simulink model "TBRe19_ECU_1_WORKING_190726"  (R2017b)
settings: Solver=FixedStepDiscrete  StartTime=0.0  StopTime=inf  FixedStep=0.0001  RelTol=1e-3
PostLoadFcn:
  | model_init();
libraries: simulink x17
(part 6 of 7)

== system TBRe19_ECU_1_WORKING_190726/MainTask/Pre_Processing_Layer/Pedal_Box/APPS and BP Plausibility ==
  note: Invert the logic so that if error is active, throttle gets multiplied by zero
  note: This block outputs the previous state from previous sample
  note: Note: This is needed by rules - including specified percentages
  note: If brake is above 20% AND accelerator is above 25%, then hold the error on until throttle is less than 5%
  note: If accelerator and brake pedal are pressed at the same time, then wait for both pedals to return to zero before sending further torque requests
  note: function [Throttle_Percentage, APPS_BP_Implausibility] = APPS_BP_Plausibility_Check(Throttle_In, Brake_In, APPS_BP_Implausibility_Prv)
      | %Plausibility check on both throttle and brake
      |
      | %Implausible case: when both brake and throttle applied
      | if (Brake_In >=20 && Throttle_In > 25)
      |     APPS_BP_Implausibility = true;
      |     Throttle_Percentage =uint8(0);
      |
      | %Implausible case: when brake pressed but throttle still not below 5%
      | elseif (APPS_BP_Implausibility_Prv && Throttle_In > 5)
      |     APPS_BP_Implausibility = true;
      |     Throttle_Percentage =uint8(0);
      |
      | %Plausible case, throttle goes below 5%
      | elseif (APPS_BP_Implausibility_Prv && Throttle_In < 5)
      |     APPS_BP_Implausibility = false;
      |     Throttle_Percentage =uint8(Throttle_In);
      |
      | %Plausible case, normal operation
      | else
      |     APPS_BP_Implausibility = false;
      |     Throttle_Percentage =uint8(Throttle_In);
      | end
  Throttle_In : Inport
  Brake_% : Inport  Port=2
  Constant : Constant  Value=20
  Constant1 : Constant  Value=25
  Constant2 : Constant  Value=5
  Logical Operator : Logic  AllPortsSameDT=off  OutDataTypeStr=boolean
  Logical Operator1 : Logic  AllPortsSameDT=off  OutDataTypeStr=boolean
  Logical Operator2 : Logic  Operator=OR  AllPortsSameDT=off  OutDataTypeStr=boolean
  Logical Operator3 : Logic  Operator=NOT  Inputs=1  AllPortsSameDT=off  OutDataTypeStr=boolean
  Product : Product  OutDataTypeStr=uint8
  Relational Operator : RelationalOperator  OutDataTypeStr=boolean  RndMeth=Simplest
  Relational Operator1 : RelationalOperator  Operator=>  OutDataTypeStr=boolean  RndMeth=Simplest
  Relational Operator2 : RelationalOperator  Operator=>  OutDataTypeStr=boolean  RndMeth=Simplest
  prv_APPS_BP1 : Delay  DelayLength=1  InitialCondition=0
  Throttle_% : Outport
  APPS_BP_Implausibility : Outport  Port=2
  wires:
  Brake_%/1 -> Relational Operator/1
  Constant/1 -> Relational Operator/2
  Constant1/1 -> Relational Operator1/2
  Constant2/1 -> Relational Operator2/2
  Throttle_In/1 -> Product/2, Relational Operator2/1, Relational Operator1/1
  prv_APPS_BP1/1 -> Logical Operator1/2
  Relational Operator2/1 -> Logical Operator1/1
  Relational Operator/1 -> Logical Operator/1
  Relational Operator1/1 -> Logical Operator/2
  Logical Operator2/1 -> APPS_BP_Implausibility/1, Logical Operator3/1, prv_APPS_BP1/1
  Logical Operator1/1 -> Logical Operator2/2
  Logical Operator/1 -> Logical Operator2/1
  Product/1 -> Throttle_%/1
  Logical Operator3/1 -> Product/1

== system TBRe19_ECU_1_WORKING_190726/MainTask/Pre_Processing_Layer/Pedal_Box/APPS_Implausibility_Check ==
  note: This sets torque to zero if APPS implausibility happens
  note: Send to CAN bus
  note: Note: 100ms is measured using 10 delays. As task runs every 10ms, 10 delays will result in a 100ms delay
  note: If the error happens continuosly for 100ms then the throttle output should be set to zero
  note: Check to see if Throttle2 is within the range of Throttle1 +/- 15%
  note: 15% is defined in rules
  note: function [APPS_Implausbility, Throttle_Percentage] = APPS_Implausibility_Check(Pedal_Sensor_Fail, Throttle1_Per, Throttle2_Per)
      | %Limit generation for comparison
      | Upper_Limit = Throttle1_Per+15;
      | Lower_Limit = Throttle1_Per-15;
      |
      | %Passes one throttle if in range and no pedal sensor errors
      | if ((Lower_Limit <= Throttle2_Per) && (Throttle2_Per <= Upper_Limit)&& Pedal_Sensor_Fail == 0)
      |     Throttle_Percentage = uint8(max(Throttle1_Per, Throttle2_Per));
      |     APPS_Implausbility = false;
      | %All other conditions result in no throttle being applied
      | else
      |     Throttle_Percentage = uint8(0);
      |     APPS_Implausbility = true;
      | end
      |
      | end
  Throttle1_Per : Inport
  Throttle2_Per : Inport  Port=2
  Constant : Constant  Value=15
  Data Type Conversion : DataTypeConversion  OutDataTypeStr=int8
  Logical Operator : Logic  Operator=OR  AllPortsSameDT=off  OutDataTypeStr=boolean
  Logical Operator3 : Logic  Operator=NOT  Inputs=1  AllPortsSameDT=off  OutDataTypeStr=boolean
  LowerLinit : Sum  Inputs=-+
  MinMax : MinMax  Inputs=2
  Product : Product
  Product of Elements : Product  Inputs=*
  Relational Operator : RelationalOperator  OutDataTypeStr=boolean  RndMeth=Simplest
  Relational Operator1 : RelationalOperator  Operator=<=  OutDataTypeStr=boolean  RndMeth=Simplest
  Tapped Delay : simulink/Discrete/Tapped Delay  vinit=0  samptime=-1  NumDelays=10  DelayOrder=Oldest  includeCurrent=off
  UpperLinit : Sum
  APPS_Implausibility : Outport
  Throttle_% : Outport  Port=2
  wires:
  Throttle1_Per/1 -> MinMax/1, UpperLinit/1, LowerLinit/2
  Throttle2_Per/1 -> MinMax/2, Relational Operator1/1, Relational Operator/1
  Logical Operator/1 -> Tapped Delay/1  "APPS_Implausibility"
  Constant/1 -> UpperLinit/2, LowerLinit/1
  UpperLinit/1 -> Relational Operator/2
  LowerLinit/1 -> Relational Operator1/2
  Relational Operator/1 -> Logical Operator/1
  Relational Operator1/1 -> Logical Operator/2
  Logical Operator3/1 -> Data Type Conversion/1
  Data Type Conversion/1 -> Product/2
  Tapped Delay/1 -> Product of Elements/1
  Product of Elements/1 -> APPS_Implausibility/1, Logical Operator3/1
  MinMax/1 -> Product/1
  Product/1 -> Throttle_%/1

== system TBRe19_ECU_1_WORKING_190726/MainTask/Pre_Processing_Layer/Pedal_Box/BPPS_Implausibility_Check ==
  note: Note: Not needed for rules
  note: Output to CAN
  note: function [APPS_Implausbility, Throttle_Percentage] = APPS_Implausibility_Check(Pedal_Sensor_Fail, Throttle1_Per, Throttle2_Per)
      | %Limit generation for comparison
      | Upper_Limit = Throttle1_Per+15;
      | Lower_Limit = Throttle1_Per-15;
      |
      | %Passes one throttle if in range and no pedal sensor errors
      | if ((Lower_Limit <= Throttle2_Per) && (Throttle2_Per <= Upper_Limit)&& Pedal_Sensor_Fail == 0)
      |     Throttle_Percentage = uint8(max(Throttle1_Per, Throttle2_Per));
      |     APPS_Implausbility = false;
      | %All other conditions result in no throttle being applied
      | else
      |     Throttle_Percentage = uint8(0);
      |     APPS_Implausbility = true;
      | end
      |
      | end
  note: If the error happens continuosly for 100ms then the throttle output should be set to zero
  note: Note: 100ms is measured using 10 delays. As task runs every 10ms, 10 delays will result in a 100ms delay
  Brake1_Per : Inport
  Brake2_Per : Inport  Port=2
  Constant : Constant  Value=15
  Logical Operator : Logic  Operator=OR  AllPortsSameDT=off  OutDataTypeStr=boolean
  LowerLinit : Sum  Inputs=-+
  MinMax : MinMax  Function=max  Inputs=2
  Product of Elements : Product  Inputs=*
  Relational Operator : RelationalOperator  OutDataTypeStr=boolean  RndMeth=Simplest
  Relational Operator1 : RelationalOperator  Operator=<=  OutDataTypeStr=boolean  RndMeth=Simplest
  Tapped Delay : simulink/Discrete/Tapped Delay  vinit=0  samptime=-1  NumDelays=10  DelayOrder=Oldest  includeCurrent=off
  UpperLinit : Sum
  Brake_% : Outport
  BPPS_Implausibility : Outport  Port=2
  wires:
  Brake1_Per/1 -> MinMax/1, UpperLinit/1, LowerLinit/2
  Brake2_Per/1 -> MinMax/2, Relational Operator1/1, Relational Operator/1
  Logical Operator/1 -> Tapped Delay/1  "APPS_Implausibility"
  Constant/1 -> UpperLinit/2, LowerLinit/1
  UpperLinit/1 -> Relational Operator/2
  LowerLinit/1 -> Relational Operator1/2
  Relational Operator/1 -> Logical Operator/1
  Relational Operator1/1 -> Logical Operator/2
  Tapped Delay/1 -> Product of Elements/1
  Product of Elements/1 -> BPPS_Implausibility/1
  MinMax/1 -> Brake_%/1

== system TBRe19_ECU_1_WORKING_190726/MainTask/Pre_Processing_Layer/Pedal_Box/Sensor Plausibility ==
  note: Check if the readings from the sensors are outside expected range
      | e.g. If a 5V sensor is giving a reading of 12V
      |
      | Note: Not needed for rules
  <Throttle1_Voltage> : Inport
  <Throttle2_Voltage> : Inport  Port=2
  <Brake_Voltage> : Inport  Port=3
  <Brake_Voltage>1 : Inport  Port=4
  <Brake_Voltage>2 : Inport  Port=5
  Sensor_Diag : MATLAB Function  TreatAsAtomicUnit=on
  Pedal_Sensor_Fail : Outport
  TV1_Out : Outport  Port=2
  TV2_Out : Outport  Port=3
  BVPot_Out : Outport  Port=4
  BV1_Out : Outport  Port=5
  BV1_Out1 : Outport  Port=6
  wires:
  <Throttle1_Voltage>/1 -> Sensor_Diag/1(TV_1)
  <Throttle2_Voltage>/1 -> Sensor_Diag/2(TV_2)
  <Brake_Voltage>/1 -> Sensor_Diag/3(BV_POT)
  Sensor_Diag/1(Pedal_Sensor_Fail) -> Pedal_Sensor_Fail/1
  Sensor_Diag/2(TV1_Out) -> TV1_Out/1
  Sensor_Diag/3(TV2_Out) -> TV2_Out/1
  Sensor_Diag/4(BVPot_Out) -> BVPot_Out/1
  <Brake_Voltage>1/1 -> Sensor_Diag/4(BV_1)
  <Brake_Voltage>2/1 -> Sensor_Diag/5(BV_2)
  Sensor_Diag/5(BV1_Out) -> BV1_Out/1
  Sensor_Diag/6(BV2_Out) -> BV1_Out1/1

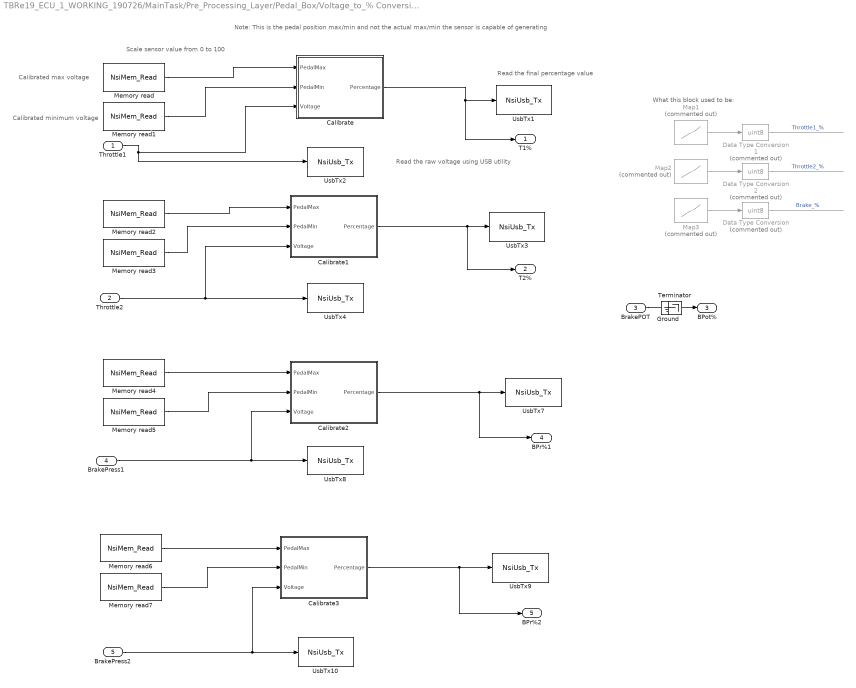
== system TBRe19_ECU_1_WORKING_190726/MainTask/Pre_Processing_Layer/Pedal_Box/Voltage_to_% Conversion ==
  note: Read the final percentage value
  note: Read the raw voltage using USB utility
  note: Note: This is the pedal position max/min and not the actual max/min the sensor is capable of generating
  note: Calibrated minimum voltage
  note: Calibrated max voltage
  note: What this block used to be:
  note: Scale sensor value from 0 to 100
  Throttle1 : Inport
  Throttle2 : Inport  Port=2
  BrakePOT : Inport  Port=3
  BrakePress1 : Inport  Port=4
  BrakePress2 : Inport  Port=5
  Calibrate : Subsystem
  Calibrate1 : Subsystem
  Calibrate2 : Subsystem
  Calibrate3 : Subsystem
  Data Type Conversion : DataTypeConversion  Commented=on  OutDataTypeStr=uint8
  Data Type Conversion1 : DataTypeConversion  Commented=on  OutDataTypeStr=uint8
  Data Type Conversion2 : DataTypeConversion  Commented=on  OutDataTypeStr=uint8
  Ground : Ground
  Map1 : Lookup_n-D  Commented=on  NumberOfTableDimensions=1  BreakpointsForDimension1=[0000,5000]  Table=[0,100]  ExtrapMethod=Clip  UseLastTableValue=on  InternalRulePriority=Speed  RndMeth=Simplest  InputSameDT=on
  Map2 : Lookup_n-D  Commented=on  NumberOfTableDimensions=1  BreakpointsForDimension1=[0000,5000]  Table=[0,100]  ExtrapMethod=Clip  UseLastTableValue=on  InternalRulePriority=Speed  RndMeth=Simplest  InputSameDT=on
  Map3 : Lookup_n-D  Commented=on  NumberOfTableDimensions=1  BreakpointsForDimension1=[2800,5600]  Table=[0,100]  ExtrapMethod=Clip  UseLastTableValue=on  InternalRulePriority=Speed  RndMeth=Simplest  InputSameDT=on
  Memory read : S-Function  FunctionName=NsiMem_Read  Parameters=name_var,type_var,size_var,tunable_var  SFunctionDeploymentMode=off  EnableBusSupport=off  mask(Memory read){name_var=Throttle1_High, type_var=Unsigned Word, size_var=1, tunable_var=on}
      mask prompts: name_var "Variable name :"; type_var "Type :"; size_var "Dim of table :"; tunable_var "Is Tunable By USB?"
      mask help: Reads current value of variable memory declared in the configurator block in calibration page.
      mask init:
      | NsiMem_Read_InitializationFcn();
      settings: OpenFcn=NsiMem_Read_OpenFcn();
      mask Help:
      | eval('block=get_param(gcb, ''RTWdata'');')
      | web([docroot '\toolbox\MUXlink\html\blocks/' block.MUXlink_BlockType '.html'])
      mask TypeOptions name_var: Gearing_Ratio | Wheel_Size | Brake1_High | Brake2_High | Throttle1_High | Throttle2_High | Brake1_Low | Brake2_Low | Throttle1_Low | Throttle2_Low | Max_Torque_Std | Max_Torque_Boost | MCU_Ignition | LV_Low_Voltage_Warning | MCUMotor_Temp_Warning | Target_Slip_Ratio | TC_P_Gain | MinTC_Torque | Max_Regen | Throttle_Active_Threshold | Brake_Active_Threshold | INV_Torque_limit | INV_Speed_Limit_Fwd | INV_Speed_limit_Rev | INV_DC_Link_Target | INV_DC_Link_Regen_Imax | INV_DC_Link_Discharge_Imax | INV_Regen_Torque_Limit | INV_Id_Debug | INV_Iq_debug | Init_System_Start | Init_System_end | Brake1_Pressure_Scaling | Brake2_Pressure_Scaling
      mask Callback name_var: NsiMem_Read_ApplyFcn(1);
      mask TypeOptions type_var: Boolean | Signed Byte | Unsigned Byte | Signed Word | Unsigned Word | Signed Double Word | Unsigned Double Word | Single Float | Double Float
      mask Callback type_var: NsiMem_Read_ApplyFcn(2);
      mask Callback size_var: NsiMem_Read_ApplyFcn(3);
      mask Callback tunable_var: NsiMem_Read_ApplyFcn(4);
      mask Display: image(imread('nsi.bmp'));text(0.5, 0.35, 'Throttle1_High', 'horizontalAlignment', 'center', 'verticalAlignment', 'base');plot([0.05 0.05 0.05 0.05 0.05 0.05 0.05 0.05 0.05 0.05]);port_label('output', 1, 'Read');
  Memory read1 : S-Function  FunctionName=NsiMem_Read  Parameters=name_var,type_var,size_var,tunable_var  SFunctionDeploymentMode=off  EnableBusSupport=off  mask(Memory read){name_var=Throttle1_Low, type_var=Unsigned Word, size_var=1, tunable_var=on}
      mask prompts: name_var "Variable name :"; type_var "Type :"; size_var "Dim of table :"; tunable_var "Is Tunable By USB?"
      mask help: Reads current value of variable memory declared in the configurator block in calibration page.
      mask init:
      | NsiMem_Read_InitializationFcn();
      settings: OpenFcn=NsiMem_Read_OpenFcn();
      mask Help:
      | eval('block=get_param(gcb, ''RTWdata'');')
      | web([docroot '\toolbox\MUXlink\html\blocks/' block.MUXlink_BlockType '.html'])
      mask TypeOptions name_var: Gearing_Ratio | Wheel_Size | Brake1_High | Brake2_High | Throttle1_High | Throttle2_High | Brake1_Low | Brake2_Low | Throttle1_Low | Throttle2_Low | Max_Torque_Std | Max_Torque_Boost | MCU_Ignition | LV_Low_Voltage_Warning | MCUMotor_Temp_Warning | Target_Slip_Ratio | TC_P_Gain | MinTC_Torque | Max_Regen | Throttle_Active_Threshold | Brake_Active_Threshold | INV_Torque_limit | INV_Speed_Limit_Fwd | INV_Speed_limit_Rev | INV_DC_Link_Target | INV_DC_Link_Regen_Imax | INV_DC_Link_Discharge_Imax | INV_Regen_Torque_Limit | INV_Id_Debug | INV_Iq_debug | Init_System_Start | Init_System_end | Brake1_Pressure_Scaling | Brake2_Pressure_Scaling
      mask Callback name_var: NsiMem_Read_ApplyFcn(1);
      mask TypeOptions type_var: Boolean | Signed Byte | Unsigned Byte | Signed Word | Unsigned Word | Signed Double Word | Unsigned Double Word | Single Float | Double Float
      mask Callback type_var: NsiMem_Read_ApplyFcn(2);
      mask Callback size_var: NsiMem_Read_ApplyFcn(3);
      mask Callback tunable_var: NsiMem_Read_ApplyFcn(4);
      mask Display: image(imread('nsi.bmp'));text(0.5, 0.35, 'Throttle1_Low', 'horizontalAlignment', 'center', 'verticalAlignment', 'base');plot([0.05 0.05 0.05 0.05 0.05 0.05 0.05 0.05 0.05 0.05]);port_label('output', 1, 'Read');
  Memory read2 : S-Function  FunctionName=NsiMem_Read  Parameters=name_var,type_var,size_var,tunable_var  SFunctionDeploymentMode=off  EnableBusSupport=off  mask(Memory read){name_var=Throttle2_High, type_var=Unsigned Word, size_var=1, tunable_var=on}
      mask prompts: name_var "Variable name :"; type_var "Type :"; size_var "Dim of table :"; tunable_var "Is Tunable By USB?"
      mask help: Reads current value of variable memory declared in the configurator block in calibration page.
      mask init:
      | NsiMem_Read_InitializationFcn();
      settings: OpenFcn=NsiMem_Read_OpenFcn();
      mask Help:
      | eval('block=get_param(gcb, ''RTWdata'');')
      | web([docroot '\toolbox\MUXlink\html\blocks/' block.MUXlink_BlockType '.html'])
      mask TypeOptions name_var: Gearing_Ratio | Wheel_Size | Brake1_High | Brake2_High | Throttle1_High | Throttle2_High | Brake1_Low | Brake2_Low | Throttle1_Low | Throttle2_Low | Max_Torque_Std | Max_Torque_Boost | MCU_Ignition | LV_Low_Voltage_Warning | MCUMotor_Temp_Warning | Target_Slip_Ratio | TC_P_Gain | MinTC_Torque | Max_Regen | Throttle_Active_Threshold | Brake_Active_Threshold | INV_Torque_limit | INV_Speed_Limit_Fwd | INV_Speed_limit_Rev | INV_DC_Link_Target | INV_DC_Link_Regen_Imax | INV_DC_Link_Discharge_Imax | INV_Regen_Torque_Limit | INV_Id_Debug | INV_Iq_debug | Init_System_Start | Init_System_end | Brake1_Pressure_Scaling | Brake2_Pressure_Scaling
      mask Callback name_var: NsiMem_Read_ApplyFcn(1);
      mask TypeOptions type_var: Boolean | Signed Byte | Unsigned Byte | Signed Word | Unsigned Word | Signed Double Word | Unsigned Double Word | Single Float | Double Float
      mask Callback type_var: NsiMem_Read_ApplyFcn(2);
      mask Callback size_var: NsiMem_Read_ApplyFcn(3);
      mask Callback tunable_var: NsiMem_Read_ApplyFcn(4);
      mask Display: image(imread('nsi.bmp'));text(0.5, 0.35, 'Throttle2_High', 'horizontalAlignment', 'center', 'verticalAlignment', 'base');plot([0.05 0.05 0.05 0.05 0.05 0.05 0.05 0.05 0.05 0.05]);port_label('output', 1, 'Read');
  Memory read3 : S-Function  FunctionName=NsiMem_Read  Parameters=name_var,type_var,size_var,tunable_var  SFunctionDeploymentMode=off  EnableBusSupport=off  mask(Memory read){name_var=Throttle2_Low, type_var=Unsigned Word, size_var=1, tunable_var=on}
      mask prompts: name_var "Variable name :"; type_var "Type :"; size_var "Dim of table :"; tunable_var "Is Tunable By USB?"
      mask help: Reads current value of variable memory declared in the configurator block in calibration page.
      mask init:
      | NsiMem_Read_InitializationFcn();
      settings: OpenFcn=NsiMem_Read_OpenFcn();
      mask Help:
      | eval('block=get_param(gcb, ''RTWdata'');')
      | web([docroot '\toolbox\MUXlink\html\blocks/' block.MUXlink_BlockType '.html'])
      mask TypeOptions name_var: Gearing_Ratio | Wheel_Size | Brake1_High | Brake2_High | Throttle1_High | Throttle2_High | Brake1_Low | Brake2_Low | Throttle1_Low | Throttle2_Low | Max_Torque_Std | Max_Torque_Boost | MCU_Ignition | LV_Low_Voltage_Warning | MCUMotor_Temp_Warning | Target_Slip_Ratio | TC_P_Gain | MinTC_Torque | Max_Regen | Throttle_Active_Threshold | Brake_Active_Threshold | INV_Torque_limit | INV_Speed_Limit_Fwd | INV_Speed_limit_Rev | INV_DC_Link_Target | INV_DC_Link_Regen_Imax | INV_DC_Link_Discharge_Imax | INV_Regen_Torque_Limit | INV_Id_Debug | INV_Iq_debug | Init_System_Start | Init_System_end | Brake1_Pressure_Scaling | Brake2_Pressure_Scaling
      mask Callback name_var: NsiMem_Read_ApplyFcn(1);
      mask TypeOptions type_var: Boolean | Signed Byte | Unsigned Byte | Signed Word | Unsigned Word | Signed Double Word | Unsigned Double Word | Single Float | Double Float
      mask Callback type_var: NsiMem_Read_ApplyFcn(2);
      mask Callback size_var: NsiMem_Read_ApplyFcn(3);
      mask Callback tunable_var: NsiMem_Read_ApplyFcn(4);
      mask Display: image(imread('nsi.bmp'));text(0.5, 0.35, 'Throttle2_Low', 'horizontalAlignment', 'center', 'verticalAlignment', 'base');plot([0.05 0.05 0.05 0.05 0.05 0.05 0.05 0.05 0.05 0.05]);port_label('output', 1, 'Read');
  Memory read4 : S-Function  FunctionName=NsiMem_Read  Parameters=name_var,type_var,size_var,tunable_var  SFunctionDeploymentMode=off  EnableBusSupport=off  mask(Memory read){name_var=Brake1_High, type_var=Unsigned Word, size_var=1, tunable_var=on}
      mask prompts: name_var "Variable name :"; type_var "Type :"; size_var "Dim of table :"; tunable_var "Is Tunable By USB?"
      mask help: Reads current value of variable memory declared in the configurator block in calibration page.
      mask init:
      | NsiMem_Read_InitializationFcn();
      settings: OpenFcn=NsiMem_Read_OpenFcn();
      mask Help:
      | eval('block=get_param(gcb, ''RTWdata'');')
      | web([docroot '\toolbox\MUXlink\html\blocks/' block.MUXlink_BlockType '.html'])
      mask TypeOptions name_var: Gearing_Ratio | Wheel_Size | Brake1_High | Brake2_High | Throttle1_High | Throttle2_High | Brake1_Low | Brake2_Low | Throttle1_Low | Throttle2_Low | Max_Torque_Std | Max_Torque_Boost | MCU_Ignition | LV_Low_Voltage_Warning | MCUMotor_Temp_Warning | Target_Slip_Ratio | TC_P_Gain | MinTC_Torque | Max_Regen | Throttle_Active_Threshold | Brake_Active_Threshold | INV_Torque_limit | INV_Speed_Limit_Fwd | INV_Speed_limit_Rev | INV_DC_Link_Target | INV_DC_Link_Regen_Imax | INV_DC_Link_Discharge_Imax | INV_Regen_Torque_Limit | INV_Id_Debug | INV_Iq_debug | Init_System_Start | Init_System_end | Brake1_Pressure_Scaling | Brake2_Pressure_Scaling
      mask Callback name_var: NsiMem_Read_ApplyFcn(1);
      mask TypeOptions type_var: Boolean | Signed Byte | Unsigned Byte | Signed Word | Unsigned Word | Signed Double Word | Unsigned Double Word | Single Float | Double Float
      mask Callback type_var: NsiMem_Read_ApplyFcn(2);
      mask Callback size_var: NsiMem_Read_ApplyFcn(3);
      mask Callback tunable_var: NsiMem_Read_ApplyFcn(4);
      mask Display: image(imread('nsi.bmp'));text(0.5, 0.35, 'Brake1_High', 'horizontalAlignment', 'center', 'verticalAlignment', 'base');plot([0.05 0.05 0.05 0.05 0.05 0.05 0.05 0.05 0.05 0.05]);port_label('output', 1, 'Read');
  Memory read5 : S-Function  FunctionName=NsiMem_Read  Parameters=name_var,type_var,size_var,tunable_var  SFunctionDeploymentMode=off  EnableBusSupport=off  mask(Memory read){name_var=Brake1_Low, type_var=Unsigned Word, size_var=1, tunable_var=on}
      mask prompts: name_var "Variable name :"; type_var "Type :"; size_var "Dim of table :"; tunable_var "Is Tunable By USB?"
      mask help: Reads current value of variable memory declared in the configurator block in calibration page.
      mask init:
      | NsiMem_Read_InitializationFcn();
      settings: OpenFcn=NsiMem_Read_OpenFcn();
      mask Help:
      | eval('block=get_param(gcb, ''RTWdata'');')
      | web([docroot '\toolbox\MUXlink\html\blocks/' block.MUXlink_BlockType '.html'])
      mask TypeOptions name_var: Gearing_Ratio | Wheel_Size | Brake1_High | Brake2_High | Throttle1_High | Throttle2_High | Brake1_Low | Brake2_Low | Throttle1_Low | Throttle2_Low | Max_Torque_Std | Max_Torque_Boost | MCU_Ignition | LV_Low_Voltage_Warning | MCUMotor_Temp_Warning | Target_Slip_Ratio | TC_P_Gain | MinTC_Torque | Max_Regen | Throttle_Active_Threshold | Brake_Active_Threshold | INV_Torque_limit | INV_Speed_Limit_Fwd | INV_Speed_limit_Rev | INV_DC_Link_Target | INV_DC_Link_Regen_Imax | INV_DC_Link_Discharge_Imax | INV_Regen_Torque_Limit | INV_Id_Debug | INV_Iq_debug | Init_System_Start | Init_System_end | Brake1_Pressure_Scaling | Brake2_Pressure_Scaling
      mask Callback name_var: NsiMem_Read_ApplyFcn(1);
      mask TypeOptions type_var: Boolean | Signed Byte | Unsigned Byte | Signed Word | Unsigned Word | Signed Double Word | Unsigned Double Word | Single Float | Double Float
      mask Callback type_var: NsiMem_Read_ApplyFcn(2);
      mask Callback size_var: NsiMem_Read_ApplyFcn(3);
      mask Callback tunable_var: NsiMem_Read_ApplyFcn(4);
      mask Display: image(imread('nsi.bmp'));text(0.5, 0.35, 'Brake1_Low', 'horizontalAlignment', 'center', 'verticalAlignment', 'base');plot([0.05 0.05 0.05 0.05 0.05 0.05 0.05 0.05 0.05 0.05]);port_label('output', 1, 'Read');
  Memory read6 : S-Function  FunctionName=NsiMem_Read  Parameters=name_var,type_var,size_var,tunable_var  SFunctionDeploymentMode=off  EnableBusSupport=off  mask(Memory read){name_var=Brake1_High, type_var=Unsigned Word, size_var=1, tunable_var=on}
      mask prompts: name_var "Variable name :"; type_var "Type :"; size_var "Dim of table :"; tunable_var "Is Tunable By USB?"
      mask help: Reads current value of variable memory declared in the configurator block in calibration page.
      mask init:
      | NsiMem_Read_InitializationFcn();
      settings: OpenFcn=NsiMem_Read_OpenFcn();
      mask Help:
      | eval('block=get_param(gcb, ''RTWdata'');')
      | web([docroot '\toolbox\MUXlink\html\blocks/' block.MUXlink_BlockType '.html'])
      mask TypeOptions name_var: Gearing_Ratio | Wheel_Size | Brake1_High | Brake2_High | Throttle1_High | Throttle2_High | Brake1_Low | Brake2_Low | Throttle1_Low | Throttle2_Low | Max_Torque_Std | Max_Torque_Boost | MCU_Ignition | LV_Low_Voltage_Warning | MCUMotor_Temp_Warning | Target_Slip_Ratio | TC_P_Gain | MinTC_Torque | Max_Regen | Throttle_Active_Threshold | Brake_Active_Threshold | INV_Torque_limit | INV_Speed_Limit_Fwd | INV_Speed_limit_Rev | INV_DC_Link_Target | INV_DC_Link_Regen_Imax | INV_DC_Link_Discharge_Imax | INV_Regen_Torque_Limit | INV_Id_Debug | INV_Iq_debug | Init_System_Start | Init_System_end | Brake1_Pressure_Scaling | Brake2_Pressure_Scaling
      mask Callback name_var: NsiMem_Read_ApplyFcn(1);
      mask TypeOptions type_var: Boolean | Signed Byte | Unsigned Byte | Signed Word | Unsigned Word | Signed Double Word | Unsigned Double Word | Single Float | Double Float
      mask Callback type_var: NsiMem_Read_ApplyFcn(2);
      mask Callback size_var: NsiMem_Read_ApplyFcn(3);
      mask Callback tunable_var: NsiMem_Read_ApplyFcn(4);
      mask Display: image(imread('nsi.bmp'));text(0.5, 0.35, 'Brake1_High', 'horizontalAlignment', 'center', 'verticalAlignment', 'base');plot([0.05 0.05 0.05 0.05 0.05 0.05 0.05 0.05 0.05 0.05]);port_label('output', 1, 'Read');
  Memory read7 : S-Function  FunctionName=NsiMem_Read  Parameters=name_var,type_var,size_var,tunable_var  SFunctionDeploymentMode=off  EnableBusSupport=off  mask(Memory read){name_var=Brake1_Low, type_var=Unsigned Word, size_var=1, tunable_var=on}
      mask prompts: name_var "Variable name :"; type_var "Type :"; size_var "Dim of table :"; tunable_var "Is Tunable By USB?"
      mask help: Reads current value of variable memory declared in the configurator block in calibration page.
      mask init:
      | NsiMem_Read_InitializationFcn();
      settings: OpenFcn=NsiMem_Read_OpenFcn();
      mask Help:
      | eval('block=get_param(gcb, ''RTWdata'');')
      | web([docroot '\toolbox\MUXlink\html\blocks/' block.MUXlink_BlockType '.html'])
      mask TypeOptions name_var: Gearing_Ratio | Wheel_Size | Brake1_High | Brake2_High | Throttle1_High | Throttle2_High | Brake1_Low | Brake2_Low | Throttle1_Low | Throttle2_Low | Max_Torque_Std | Max_Torque_Boost | MCU_Ignition | LV_Low_Voltage_Warning | MCUMotor_Temp_Warning | Target_Slip_Ratio | TC_P_Gain | MinTC_Torque | Max_Regen | Throttle_Active_Threshold | Brake_Active_Threshold | INV_Torque_limit | INV_Speed_Limit_Fwd | INV_Speed_limit_Rev | INV_DC_Link_Target | INV_DC_Link_Regen_Imax | INV_DC_Link_Discharge_Imax | INV_Regen_Torque_Limit | INV_Id_Debug | INV_Iq_debug | Init_System_Start | Init_System_end | Brake1_Pressure_Scaling | Brake2_Pressure_Scaling
      mask Callback name_var: NsiMem_Read_ApplyFcn(1);
      mask TypeOptions type_var: Boolean | Signed Byte | Unsigned Byte | Signed Word | Unsigned Word | Signed Double Word | Unsigned Double Word | Single Float | Double Float
      mask Callback type_var: NsiMem_Read_ApplyFcn(2);
      mask Callback size_var: NsiMem_Read_ApplyFcn(3);
      mask Callback tunable_var: NsiMem_Read_ApplyFcn(4);
      mask Display: image(imread('nsi.bmp'));text(0.5, 0.35, 'Brake1_Low', 'horizontalAlignment', 'center', 'verticalAlignment', 'base');plot([0.05 0.05 0.05 0.05 0.05 0.05 0.05 0.05 0.05 0.05]);port_label('output', 1, 'Read');
  Terminator : Terminator
  UsbTx1 : S-Function  FunctionName=NsiUsb_Tx  Parameters=signame,resolution,offset,unite  SFunctionDeploymentMode=off  EnableBusSupport=off  mask(MUXlink Usb Tx){signame=Throttle1Pec, resolution=1, offset=0, unite=%}
      mask prompts: signame "Signal name ?"; resolution "Resolution ?"; offset "Offset ?"; unite "Unit ?"
      mask help: Transmit a frame on the USB Channel.
      mask init:
      | NsiUsb_Tx_InitializationFcn();
      settings: OpenFcn=NsiUsb_Tx_OpenFcn();
      mask Help:
      | eval('block=get_param(gcb, ''RTWdata'');')
      | web([docroot '\toolbox\MUXlink\html\blocks/' block.MUXlink_BlockType '.html'])
      mask Callback signame: NsiUsb_Tx_ApplyFcn(1);
      mask Callback resolution: NsiUsb_Tx_ApplyFcn(2);
      mask Callback offset: NsiUsb_Tx_ApplyFcn(3);
      mask Callback unite: NsiUsb_Tx_ApplyFcn(4);
      mask Display: image(imread('nsi.bmp'));text(0.5, 0.2, 'USB Tx', 'horizontalAlignment', 'center', 'verticalAlignment', 'base');plot([0.05 0.05 0.05 0.05 0.05 0.05 0.05 0.05 0.05 0.05]);port_label('input',1, 'Throttle1Pec');
  UsbTx10 : S-Function  FunctionName=NsiUsb_Tx  Parameters=signame,resolution,offset,unite  SFunctionDeploymentMode=off  EnableBusSupport=off  mask(MUXlink Usb Tx){signame=Brake2V, resolution=1, offset=0, unite=mV}
      mask prompts: signame "Signal name ?"; resolution "Resolution ?"; offset "Offset ?"; unite "Unit ?"
      mask help: Transmit a frame on the USB Channel.
      mask init:
      | NsiUsb_Tx_InitializationFcn();
      settings: OpenFcn=NsiUsb_Tx_OpenFcn();
      mask Help:
      | eval('block=get_param(gcb, ''RTWdata'');')
      | web([docroot '\toolbox\MUXlink\html\blocks/' block.MUXlink_BlockType '.html'])
      mask Callback signame: NsiUsb_Tx_ApplyFcn(1);
      mask Callback resolution: NsiUsb_Tx_ApplyFcn(2);
      mask Callback offset: NsiUsb_Tx_ApplyFcn(3);
      mask Callback unite: NsiUsb_Tx_ApplyFcn(4);
      mask Display: image(imread('nsi.bmp'));text(0.5, 0.2, 'USB Tx', 'horizontalAlignment', 'center', 'verticalAlignment', 'base');plot([0.05 0.05 0.05 0.05 0.05 0.05 0.05 0.05 0.05 0.05]);port_label('input',1, 'Brake2V');
  UsbTx2 : S-Function  FunctionName=NsiUsb_Tx  Parameters=signame,resolution,offset,unite  SFunctionDeploymentMode=off  EnableBusSupport=off  mask(MUXlink Usb Tx){signame=Throttle1V, resolution=1, offset=0, unite=mV}
      mask prompts: signame "Signal name ?"; resolution "Resolution ?"; offset "Offset ?"; unite "Unit ?"
      mask help: Transmit a frame on the USB Channel.
      mask init:
      | NsiUsb_Tx_InitializationFcn();
      settings: OpenFcn=NsiUsb_Tx_OpenFcn();
      mask Help:
      | eval('block=get_param(gcb, ''RTWdata'');')
      | web([docroot '\toolbox\MUXlink\html\blocks/' block.MUXlink_BlockType '.html'])
      mask Callback signame: NsiUsb_Tx_ApplyFcn(1);
      mask Callback resolution: NsiUsb_Tx_ApplyFcn(2);
      mask Callback offset: NsiUsb_Tx_ApplyFcn(3);
      mask Callback unite: NsiUsb_Tx_ApplyFcn(4);
      mask Display: image(imread('nsi.bmp'));text(0.5, 0.2, 'USB Tx', 'horizontalAlignment', 'center', 'verticalAlignment', 'base');plot([0.05 0.05 0.05 0.05 0.05 0.05 0.05 0.05 0.05 0.05]);port_label('input',1, 'Throttle1V');
  UsbTx3 : S-Function  FunctionName=NsiUsb_Tx  Parameters=signame,resolution,offset,unite  SFunctionDeploymentMode=off  EnableBusSupport=off  mask(MUXlink Usb Tx){signame=Throttle2Pec, resolution=1, offset=0, unite=%}
      mask prompts: signame "Signal name ?"; resolution "Resolution ?"; offset "Offset ?"; unite "Unit ?"
      mask help: Transmit a frame on the USB Channel.
      mask init:
      | NsiUsb_Tx_InitializationFcn();
      settings: OpenFcn=NsiUsb_Tx_OpenFcn();
      mask Help:
      | eval('block=get_param(gcb, ''RTWdata'');')
      | web([docroot '\toolbox\MUXlink\html\blocks/' block.MUXlink_BlockType '.html'])
      mask Callback signame: NsiUsb_Tx_ApplyFcn(1);
      mask Callback resolution: NsiUsb_Tx_ApplyFcn(2);
      mask Callback offset: NsiUsb_Tx_ApplyFcn(3);
      mask Callback unite: NsiUsb_Tx_ApplyFcn(4);
      mask Display: image(imread('nsi.bmp'));text(0.5, 0.2, 'USB Tx', 'horizontalAlignment', 'center', 'verticalAlignment', 'base');plot([0.05 0.05 0.05 0.05 0.05 0.05 0.05 0.05 0.05 0.05]);port_label('input',1, 'Throttle2Pec');
  UsbTx4 : S-Function  FunctionName=NsiUsb_Tx  Parameters=signame,resolution,offset,unite  SFunctionDeploymentMode=off  EnableBusSupport=off  mask(MUXlink Usb Tx){signame=Throttle2V, resolution=1, offset=0, unite=mV}
      mask prompts: signame "Signal name ?"; resolution "Resolution ?"; offset "Offset ?"; unite "Unit ?"
      mask help: Transmit a frame on the USB Channel.
      mask init:
      | NsiUsb_Tx_InitializationFcn();
      settings: OpenFcn=NsiUsb_Tx_OpenFcn();
      mask Help:
      | eval('block=get_param(gcb, ''RTWdata'');')
      | web([docroot '\toolbox\MUXlink\html\blocks/' block.MUXlink_BlockType '.html'])
      mask Callback signame: NsiUsb_Tx_ApplyFcn(1);
      mask Callback resolution: NsiUsb_Tx_ApplyFcn(2);
      mask Callback offset: NsiUsb_Tx_ApplyFcn(3);
      mask Callback unite: NsiUsb_Tx_ApplyFcn(4);
      mask Display: image(imread('nsi.bmp'));text(0.5, 0.2, 'USB Tx', 'horizontalAlignment', 'center', 'verticalAlignment', 'base');plot([0.05 0.05 0.05 0.05 0.05 0.05 0.05 0.05 0.05 0.05]);port_label('input',1, 'Throttle2V');
  UsbTx7 : S-Function  FunctionName=NsiUsb_Tx  Parameters=signame,resolution,offset,unite  SFunctionDeploymentMode=off  EnableBusSupport=off  mask(MUXlink Usb Tx){signame=Brake1Pec, resolution=1, offset=0, unite=%}
      mask prompts: signame "Signal name ?"; resolution "Resolution ?"; offset "Offset ?"; unite "Unit ?"
      mask help: Transmit a frame on the USB Channel.
      mask init:
      | NsiUsb_Tx_InitializationFcn();
      settings: OpenFcn=NsiUsb_Tx_OpenFcn();
      mask Help:
      | eval('block=get_param(gcb, ''RTWdata'');')
      | web([docroot '\toolbox\MUXlink\html\blocks/' block.MUXlink_BlockType '.html'])
      mask Callback signame: NsiUsb_Tx_ApplyFcn(1);
      mask Callback resolution: NsiUsb_Tx_ApplyFcn(2);
      mask Callback offset: NsiUsb_Tx_ApplyFcn(3);
      mask Callback unite: NsiUsb_Tx_ApplyFcn(4);
      mask Display: image(imread('nsi.bmp'));text(0.5, 0.2, 'USB Tx', 'horizontalAlignment', 'center', 'verticalAlignment', 'base');plot([0.05 0.05 0.05 0.05 0.05 0.05 0.05 0.05 0.05 0.05]);port_label('input',1, 'Brake1Pec');
  UsbTx8 : S-Function  FunctionName=NsiUsb_Tx  Parameters=signame,resolution,offset,unite  SFunctionDeploymentMode=off  EnableBusSupport=off  mask(MUXlink Usb Tx){signame=Brake1V, resolution=1, offset=0, unite=mV}
      mask prompts: signame "Signal name ?"; resolution "Resolution ?"; offset "Offset ?"; unite "Unit ?"
      mask help: Transmit a frame on the USB Channel.
      mask init:
      | NsiUsb_Tx_InitializationFcn();
      settings: OpenFcn=NsiUsb_Tx_OpenFcn();
      mask Help:
      | eval('block=get_param(gcb, ''RTWdata'');')
      | web([docroot '\toolbox\MUXlink\html\blocks/' block.MUXlink_BlockType '.html'])
      mask Callback signame: NsiUsb_Tx_ApplyFcn(1);
      mask Callback resolution: NsiUsb_Tx_ApplyFcn(2);
      mask Callback offset: NsiUsb_Tx_ApplyFcn(3);
      mask Callback unite: NsiUsb_Tx_ApplyFcn(4);
      mask Display: image(imread('nsi.bmp'));text(0.5, 0.2, 'USB Tx', 'horizontalAlignment', 'center', 'verticalAlignment', 'base');plot([0.05 0.05 0.05 0.05 0.05 0.05 0.05 0.05 0.05 0.05]);port_label('input',1, 'Brake1V');
  UsbTx9 : S-Function  FunctionName=NsiUsb_Tx  Parameters=signame,resolution,offset,unite  SFunctionDeploymentMode=off  EnableBusSupport=off  mask(MUXlink Usb Tx){signame=Brake2Pec, resolution=1, offset=0, unite=%}
      mask prompts: signame "Signal name ?"; resolution "Resolution ?"; offset "Offset ?"; unite "Unit ?"
      mask help: Transmit a frame on the USB Channel.
      mask init:
      | NsiUsb_Tx_InitializationFcn();
      settings: OpenFcn=NsiUsb_Tx_OpenFcn();
      mask Help:
      | eval('block=get_param(gcb, ''RTWdata'');')
      | web([docroot '\toolbox\MUXlink\html\blocks/' block.MUXlink_BlockType '.html'])
      mask Callback signame: NsiUsb_Tx_ApplyFcn(1);
      mask Callback resolution: NsiUsb_Tx_ApplyFcn(2);
      mask Callback offset: NsiUsb_Tx_ApplyFcn(3);
      mask Callback unite: NsiUsb_Tx_ApplyFcn(4);
      mask Display: image(imread('nsi.bmp'));text(0.5, 0.2, 'USB Tx', 'horizontalAlignment', 'center', 'verticalAlignment', 'base');plot([0.05 0.05 0.05 0.05 0.05 0.05 0.05 0.05 0.05 0.05]);port_label('input',1, 'Brake2Pec');
  T1% : Outport
  T2% : Outport  Port=2
  BPot% : Outport  Port=3
  BPr%1 : Outport  Port=4
  BPr%2 : Outport  Port=5
  wires:
  ? -> Map1/1
  Data Type Conversion1/1 -> ?  "Throttle1_%"
  Map1/1 -> Data Type Conversion1/1
  Throttle1/1 -> Calibrate/3(Voltage), UsbTx2/1
  Data Type Conversion2/1 -> ?  "Throttle2_%"
  ? -> Map2/1
  Map3/1 -> Data Type Conversion/1
  ? -> Map3/1
  Data Type Conversion/1 -> ?  "Brake_%"
  Map2/1 -> Data Type Conversion2/1
  Memory read3/1 -> Calibrate1/2(PedalMin)
  Throttle2/1 -> Calibrate1/3(Voltage), UsbTx4/1
  BrakePress1/1 -> UsbTx8/1, Calibrate2/3(Voltage)
  Memory read5/1 -> Calibrate2/2(PedalMin)
  BrakePress2/1 -> Calibrate3/3(Voltage), UsbTx10/1
  Calibrate/1(Percentage) -> T1%/1, UsbTx1/1
  Memory read/1 -> Calibrate/1(PedalMax)
  Memory read1/1 -> Calibrate/2(PedalMin)
  Memory read2/1 -> Calibrate1/1(PedalMax)
  Calibrate1/1(Percentage) -> T2%/1, UsbTx3/1
  Memory read4/1 -> Calibrate2/1(PedalMax)
  Calibrate2/1(Percentage) -> BPr%1/1, UsbTx7/1
  Memory read6/1 -> Calibrate3/1(PedalMax)
  Calibrate3/1(Percentage) -> BPr%2/1, UsbTx9/1
  BrakePOT/1 -> Terminator/1
  Ground/1 -> BPot%/1
  Memory read7/1 -> Calibrate3/2(PedalMin)

== system TBRe19_ECU_1_WORKING_190726/MainTask/Vehicle_Functionality_Layer/Drive_Function/OverPowerProtection ==
  note: This is also limited in the MCU
  PrePLData : Inport
  80kW with 88% efficentlcy : Constant  Value=70  OutDataTypeStr=Inherit: Inherit via back propagation
  Bus Selector : BusSelector  OutputSignals=DAL_Data.DAL_CAN.DAL_MCUCAN.Motor_Speed,DAL_Data.DAL_CAN.DAL_BMSCAN.Instant_Pack_Voltage,DAL_Data.DAL_CAN.DAL_BMSCAN.Pack_Current
  Constant : Constant  Value=9548  OutDataTypeStr=uint16
  Divide : Product  Inputs=**/  OutDataTypeStr=uint16
  Divide1 : Product  Inputs=**  OutDataTypeStr=uint16
  MinMax1 : MinMax  Function=max  Inputs=2  OutDataTypeStr=uint16
  Power : simulink/Logic and Bit Operations/Compare To Constant  relop=>=  const=75  OutDataTypeStr=boolean
  infProtection : Constant
  Max_Torque : Outport
  wires:
  Constant/1 -> Divide/1
  Divide/1 -> Max_Torque/1  "MaxTorque"
  MinMax1/1 -> Divide/3
  80kW with 88% efficentlcy/1 -> Divide/2
  infProtection/1 -> MinMax1/2
  PrePLData/1 -> Bus Selector/1
  Bus Selector/1 -> MinMax1/1  "<Motor_Speed>"
  Bus Selector/2 -> Divide1/1  "<Instant_Pack_Voltage>"
  Bus Selector/3 -> Divide1/2  "<Pack_Current>"
  Divide1/1 -> Power/1  "Power"

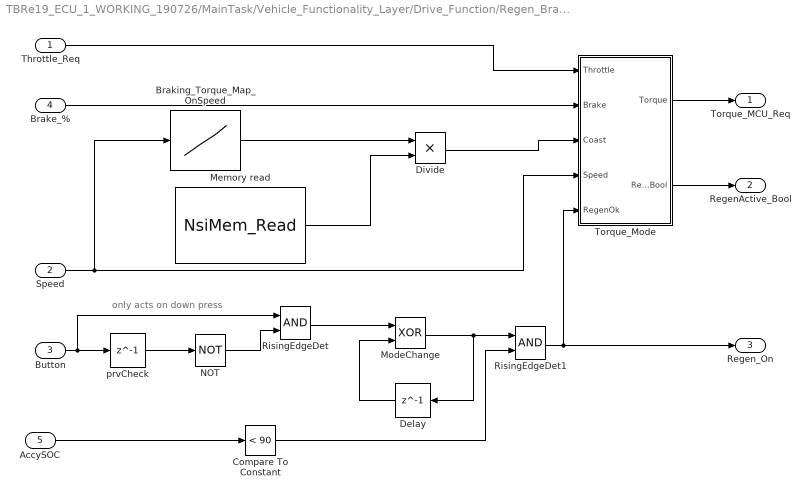
== system TBRe19_ECU_1_WORKING_190726/MainTask/Vehicle_Functionality_Layer/Drive_Function/Regen_Braking1 ==
  note: only acts on down press
  Throttle_Req : Inport
  Speed : Inport  Port=2
  Button : Inport  Port=3
  Brake_% : Inport  Port=4
  AccySOC : Inport  Port=5
  Braking_Torque_Map_OnSpeed : Lookup_n-D  NumberOfTableDimensions=1  BreakpointsForDimension1=[0,1.5,40,255]  Table=[0,0,-1,-1]  ExtrapMethod=Clip  UseLastTableValue=on  InternalRulePriority=Speed  OutDataTypeStr=double  RndMeth=Simplest  InputSameDT=on
  Compare To Constant : simulink/Logic and Bit Operations/Compare To Constant  relop=<  const=90  OutDataTypeStr=boolean
  Delay : Delay  DelayLength=1  InitialCondition=0
  Divide : Product  OutDataTypeStr=int16
  Memory read : S-Function  FunctionName=NsiMem_Read  Parameters=name_var,type_var,size_var,tunable_var  SFunctionDeploymentMode=off  EnableBusSupport=off  mask(Memory read){name_var=Max_Regen, type_var=Unsigned Byte, size_var=1, tunable_var=on}
      mask prompts: name_var "Variable name :"; type_var "Type :"; size_var "Dim of table :"; tunable_var "Is Tunable By USB?"
      mask help: Reads current value of variable memory declared in the configurator block in calibration page.
      mask init:
      | NsiMem_Read_InitializationFcn();
      settings: OpenFcn=NsiMem_Read_OpenFcn();
      mask Help:
      | eval('block=get_param(gcb, ''RTWdata'');')
      | web([docroot '\toolbox\MUXlink\html\blocks/' block.MUXlink_BlockType '.html'])
      mask TypeOptions name_var: Gearing_Ratio | Wheel_Size | Brake1_High | Brake2_High | Accel1_High | Accel2_High | Brake1_Low | Brake2_Low | Accel1_Low | Accel2_Low | Max_Torque_Std | Max_Torque_Boost | MCU_Ignition | LV_Low_Voltage_Warning | MCUMotor_Temp_Warning | Target_Slip_Ratio | TC_P_Gain | MinTC_Torque | Max_Regen
      mask Callback name_var: NsiMem_Read_ApplyFcn(1);
      mask TypeOptions type_var: Boolean | Signed Byte | Unsigned Byte | Signed Word | Unsigned Word | Signed Double Word | Unsigned Double Word | Single Float | Double Float
      mask Callback type_var: NsiMem_Read_ApplyFcn(2);
      mask Callback size_var: NsiMem_Read_ApplyFcn(3);
      mask Callback tunable_var: NsiMem_Read_ApplyFcn(4);
      mask Display: image(imread('nsi.bmp'));text(0.5, 0.35, 'Max_Regen', 'horizontalAlignment', 'center', 'verticalAlignment', 'base');plot([0.05 0.05 0.05 0.05 0.05 0.05 0.05 0.05 0.05 0.05]);port_label('output', 1, 'Read');
  ModeChange : Logic  Operator=XOR  AllPortsSameDT=off  OutDataTypeStr=boolean
  NOT : Logic  Operator=NOT  AllPortsSameDT=off  OutDataTypeStr=boolean
  RisingEdgeDet : Logic  AllPortsSameDT=off  OutDataTypeStr=boolean
  RisingEdgeDet1 : Logic  AllPortsSameDT=off  OutDataTypeStr=boolean
  Torque_Mode : MATLAB Function  TreatAsAtomicUnit=on
  prvCheck : Delay  DelayLength=1  InitialCondition=0
  Torque_MCU_Req : Outport
  RegenActive_Bool : Outport  Port=2
  Regen_On : Outport  Port=3
  wires:
  Speed/1 -> Torque_Mode/4(Speed), Braking_Torque_Map_OnSpeed/1
  Torque_Mode/1(Torque) -> Torque_MCU_Req/1
  Throttle_Req/1 -> Torque_Mode/1(Throttle)
  Torque_Mode/2(RegenBool) -> RegenActive_Bool/1
  Braking_Torque_Map_OnSpeed/1 -> Divide/1
  Brake_%/1 -> Torque_Mode/2(Brake)
  RisingEdgeDet/1 -> ModeChange/1
  NOT/1 -> RisingEdgeDet/2
  prvCheck/1 -> NOT/1
  Delay/1 -> ModeChange/2
  Button/1 -> RisingEdgeDet/1, prvCheck/1
  ModeChange/1 -> RisingEdgeDet1/1, Delay/1
  AccySOC/1 -> Compare To Constant/1
  Compare To Constant/1 -> RisingEdgeDet1/2
  RisingEdgeDet1/1 -> Regen_On/1, Torque_Mode/5(RegenOk)
  Memory read/1 -> Divide/2
  Divide/1 -> Torque_Mode/3(Coast)

== system TBRe19_ECU_1_WORKING_190726/MainTask/Vehicle_Functionality_Layer/Drive_Function/Regen_Braking_Old ==
  Throttle_Req : Inport
  Braking_% : Inport  Port=2
  Speed : Inport  Port=3
  RegenOk : Inport  Port=4
  Braking_Torque_Map_OnBrake_Max30 : Lookup_n-D  NumberOfTableDimensions=1  BreakpointsForDimension1=[0,50,70,90,100]  Table=[0,-30,-30,0,0]  ExtrapMethod=Clip  UseLastTableValue=on  InternalRulePriority=Speed  OutDataTypeStr=int16  RndMeth=Simplest  InputSameDT=on
  Coasting Brake : Constant  Value=-10  OutDataTypeStr=int16
  Torque_Mode : MATLAB Function  TreatAsAtomicUnit=on
  Torque_MCU_Req : Outport
  Regen_Bool : Outport  Port=2
  wires:
  Coasting Brake/1 -> Torque_Mode/3(Coast)
  Braking_%/1 -> Braking_Torque_Map_OnBrake_Max30/1
  Torque_Mode/1(Torque) -> Torque_MCU_Req/1
  Throttle_Req/1 -> Torque_Mode/1(Throttle)
  Speed/1 -> Torque_Mode/4(Speed)
  Braking_Torque_Map_OnBrake_Max30/1 -> Torque_Mode/2(Brake)
  RegenOk/1 -> Torque_Mode/5(RegenOk)
  Torque_Mode/2(RegenBool) -> Regen_Bool/1

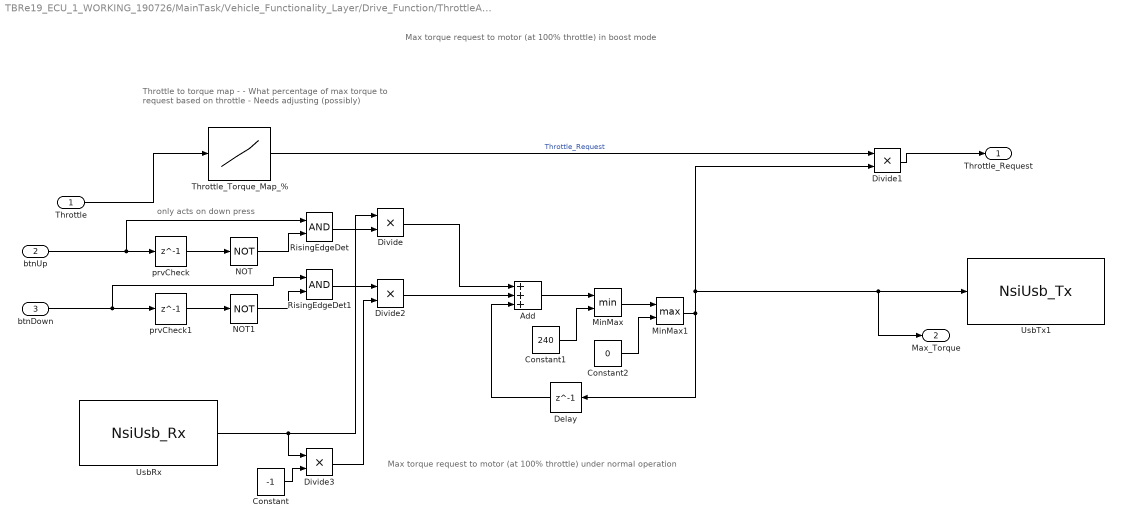
== system TBRe19_ECU_1_WORKING_190726/MainTask/Vehicle_Functionality_Layer/Drive_Function/ThrottleAddSubTorque ==
  note: Throttle to torque map -
      | - What percentage of max torque to request based on throttle
      | - Needs adjusting (possibly)
  note: Max torque request to motor (at 100% throttle) under normal operation
  note: Max torque request to motor (at 100% throttle) in boost mode
  note: only acts on down press
  Throttle : Inport
  btnUp : Inport  Port=2
  btnDown : Inport  Port=3
  Add : Sum  Inputs=+++
  Constant : Constant  Value=-1
  Constant1 : Constant  Value=240
  Constant2 : Constant  Value=0
  Delay : Delay  DelayLength=1  InitialCondition=100
  Divide{,1..3} (4 alike) : Product  Inputs=**
  MinMax : MinMax  Inputs=2
  MinMax1 : MinMax  Function=max  Inputs=2
  NOT : Logic  Operator=NOT  AllPortsSameDT=off  OutDataTypeStr=boolean
  NOT1 : Logic  Operator=NOT  AllPortsSameDT=off  OutDataTypeStr=boolean
  RisingEdgeDet : Logic  AllPortsSameDT=off  OutDataTypeStr=boolean
  RisingEdgeDet1 : Logic  AllPortsSameDT=off  OutDataTypeStr=boolean
  Throttle_Torque_Map_% : Lookup_n-D  NumberOfTableDimensions=1  BreakpointsForDimension1=[0,30,75,100]  Table=[0,5,50,100]  ExtrapMethod=Clip  UseLastTableValue=on  InternalRulePriority=Speed  OutDataTypeStr=int16  RndMeth=Simplest  InputSameDT=on
  UsbRx : S-Function  FunctionName=NsiUsb_Rx  Parameters=signame,sigtype,resolution,offset,unite,value,is_trigger  SFunctionDeploymentMode=off  EnableBusSupport=off  mask(MUXlink Usb Rx){signame=TorqueStepSize, sigtype=Unsigned Word, resolution=1, offset=0, unite=Nm, value=15, is_trigger=off}
      mask prompts: signame "Signal name :"; sigtype "Signal type :"; resolution "Resolution :"; offset "Offset :"; unite "Unit :"; value "Default value :"; is_trigger "Is trigger ?"
      mask help: Receive a frame on the USB Channel.
      mask init:
      | NsiUsb_Rx_InitializationFcn();
      settings: OpenFcn=NsiUsb_Rx_OpenFcn();
      mask Help:
      | eval('block=get_param(gcb, ''RTWdata'');')
      | web([docroot '\toolbox\MUXlink\html\blocks/' block.MUXlink_BlockType '.html'])
      mask Callback signame: NsiUsb_Rx_ApplyFcn(1);
      mask TypeOptions sigtype: Boolean | Signed Byte | Unsigned Byte | Signed Word | Unsigned Word | Signed Double Word | Unsigned Double Word | Single Float | Double Float
      mask Callback sigtype: NsiUsb_Rx_ApplyFcn(2);
      mask Callback resolution: NsiUsb_Rx_ApplyFcn(3);
      mask Callback offset: NsiUsb_Rx_ApplyFcn(4);
      mask Callback unite: NsiUsb_Rx_ApplyFcn(5);
      mask Callback value: NsiUsb_Rx_ApplyFcn(6);
      mask Callback is_trigger: NsiUsb_Rx_ApplyFcn(7);
      mask Display: image(imread('nsi.bmp'));text(0.5, 0.2, 'USB Rx', 'horizontalAlignment', 'center', 'verticalAlignment', 'base');plot([0.05 0.05 0.05 0.05 0.05 0.05 0.05 0.05 0.05 0.05]);port_label('output',1, 'TorqueStepSize');
  UsbTx1 : S-Function  FunctionName=NsiUsb_Tx  Parameters=signame,resolution,offset,unite  SFunctionDeploymentMode=off  EnableBusSupport=off  mask(MUXlink Usb Tx){signame=MaxTorque, resolution=1, offset=0, unite=km/h}
      mask prompts: signame "Signal name ?"; resolution "Resolution ?"; offset "Offset ?"; unite "Unit ?"
      mask help: Transmit a frame on the USB Channel.
      mask init:
      | NsiUsb_Tx_InitializationFcn();
      settings: OpenFcn=NsiUsb_Tx_OpenFcn();
      mask Help:
      | eval('block=get_param(gcb, ''RTWdata'');')
      | web([docroot '\toolbox\MUXlink\html\blocks/' block.MUXlink_BlockType '.html'])
      mask Callback signame: NsiUsb_Tx_ApplyFcn(1);
      mask Callback resolution: NsiUsb_Tx_ApplyFcn(2);
      mask Callback offset: NsiUsb_Tx_ApplyFcn(3);
      mask Callback unite: NsiUsb_Tx_ApplyFcn(4);
      mask Display: image(imread('nsi.bmp'));text(0.5, 0.2, 'USB Tx', 'horizontalAlignment', 'center', 'verticalAlignment', 'base');plot([0.05 0.05 0.05 0.05 0.05 0.05 0.05 0.05 0.05 0.05]);port_label('input',1, 'MaxTorque');
  prvCheck : Delay  DelayLength=1  InitialCondition=0
  prvCheck1 : Delay  DelayLength=1  InitialCondition=0
  Throttle_Request : Outport
  Max_Torque : Outport  Port=2
  wires:
  Throttle/1 -> Throttle_Torque_Map_%/1
  Throttle_Torque_Map_%/1 -> Divide1/1  "Throttle_Request"
  Divide1/1 -> Throttle_Request/1
  prvCheck/1 -> NOT/1
  NOT/1 -> RisingEdgeDet/2
  btnUp/1 -> RisingEdgeDet/1, prvCheck/1
  Add/1 -> MinMax/1
  NOT1/1 -> RisingEdgeDet1/2
  prvCheck1/1 -> NOT1/1
  btnDown/1 -> RisingEdgeDet1/1, prvCheck1/1
  RisingEdgeDet/1 -> Divide/2
  RisingEdgeDet1/1 -> Divide2/1
  UsbRx/1 -> Divide3/1, Divide/1
  Divide/1 -> Add/1
  Divide2/1 -> Add/2
  Divide3/1 -> Divide2/2
  Constant/1 -> Divide3/2
  Delay/1 -> Add/3
  MinMax/1 -> MinMax1/1
  MinMax1/1 -> Divide1/2, Max_Torque/1, UsbTx1/1, Delay/1
  Constant1/1 -> MinMax/2
  Constant2/1 -> MinMax1/2
